simulink model "zehlicka"  (R2018a)
settings: Solver=FixedStepAuto  StartTime=0.0  StopTime=1000  FixedStep=0.01  RelTol=1e-3
libraries: simulink x1
settings Model: Creator=vejvarm  LastModifiedBy=vejvarm

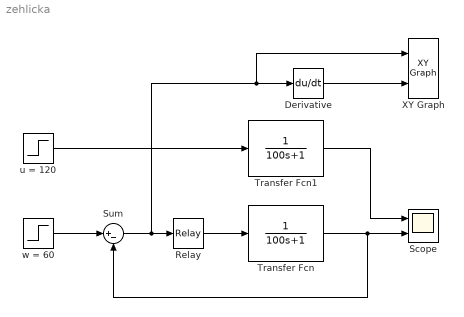
== system zehlicka ==
  Derivative : Derivative
  Relay : Relay  OnSwitchValue=5  OffSwitchValue=-5  OnOutputValue=120
  Scope : Scope  NumInputPorts=2
  Sum : Sum  Inputs=|+-
  Transfer Fcn : TransferFcn  Numerator=1  Denominator=[100 1]
  Transfer Fcn1 : TransferFcn  Numerator=1  Denominator=[100 1]
  XY Graph : simulink/Sinks/XY Graph  xmin=-inf  xmax=inf  ymin=-inf  ymax=inf  st=-1
  "u = 120 " : Step  Time=0  After=120  SampleTime=0
  w = 60 : Step  Time=0  After=60  SampleTime=0
  wires:
  Relay/1 -> Transfer Fcn/1
  Sum/1 -> XY Graph/1, Derivative/1, Relay/1
  w = 60/1 -> Sum/1
  Transfer Fcn/1 -> Sum/2, Scope/2
  Transfer Fcn1/1 -> Scope/1
  Derivative/1 -> XY Graph/2
  "u = 120 "/1 -> Transfer Fcn1/1
